simulink model "q3_1"  (R2026a)
settings: Solver=VariableStepAuto  StopTime=1
undefined symbols (not defined in the file): DiscIntNeverNeededParam
libraries: dspstat3 x4, dspfdesign x3, dspmathops x2, dspsrcs4 x1
settings Model: Creator=steve  LastModifiedBy=steve

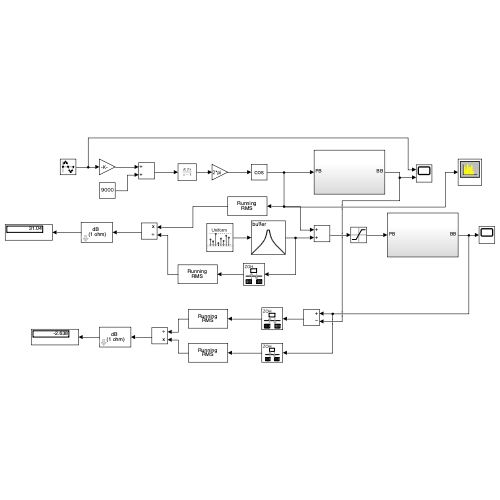
[thumbnail: Simulink's stored preview of the top-level diagram]
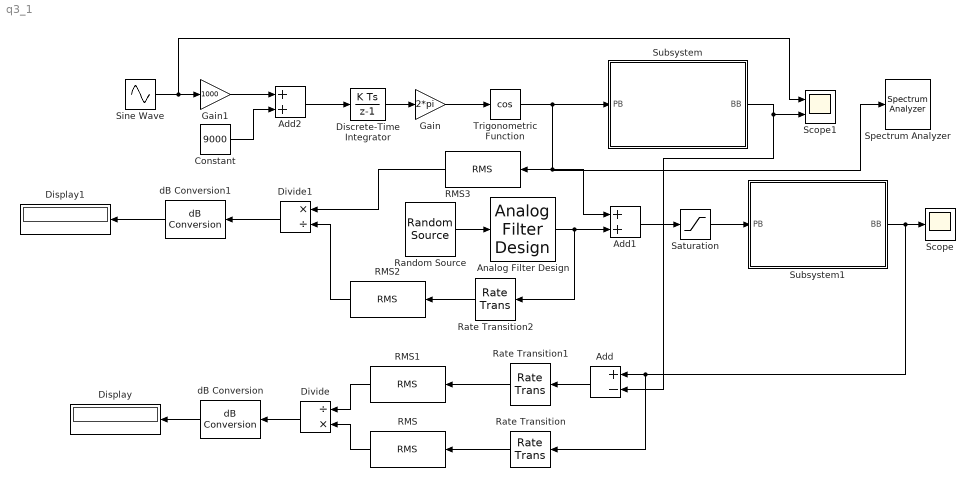
== system q3_1 ==
  Add : Sum  Inputs=+-
  Add1 : Sum
  Add2 : Sum
  Analog Filter Design : dspfdesign/Analog Filter Design  method=Butterworth  filttype=Bandpass  N=8  Wlo=8000*2*pi  Whi=10000*2*pi  Rp=2  Rs=40
  Constant : Constant  Value=9000
  Discrete-Time Integrator : DiscreteIntegrator  SampleTime=1e-5  ICPrevOutput=DiscIntNeverNeededParam  ICPrevScaledInput=DiscIntNeverNeededParam
  Display : Display
  Display1 : Display
  Divide : Product  Inputs=/*
  Divide1 : Product  Inputs=*/
  Gain : Gain  Gain=2*pi
  Gain1 : Gain  Gain=1000
  RMS{,1..3} (4 alike) : dspstat3/RMS  run=on  directionMode=Each column  dimension=1  InputProcessing=Columns as channels (frame based)  reset_popup=None
  Random Source : dspsrcs4/Random Source  SrcType=Gaussian  MinVal=0  MaxVal=1  MeanVal=0  VarVal=1e-2  RepMode=Specify seed  rawSeed=1  IsInherit=off  SampTime=1e-5  SampFrame=1  OutComplex=Real  DataType=double  SimulateUsing=Interpreted execution
  Rate Transition : RateTransition  OutPortSampleTime=1e-5
  Rate Transition1 : RateTransition  OutPortSampleTime=1e-5
  Rate Transition2 : RateTransition  OutPortSampleTime=1e-5
  Saturation : Saturate  UpperLimit=1  LowerLimit=-1
  Scope : Scope
  Scope1 : Scope  NumInputPorts=2
  Sine Wave : Sin  SineType=Sample based  Samples=1000  SampleTime=1e-5
  Spectrum Analyzer : SpectrumAnalyzer  WindowPosition=[1.000000,65.000000,1470.000000,826.000000,]  ScopeFrameLocation=window  WindowInvariantSamplesPerUpdate=on  YLimits=[-89.9778 31.3294]
  Subsystem : Subsystem
  Subsystem1 : Subsystem
  Trigonometric Function : Trigonometry  Operator=cos
  dB Conversion : dspmathops/dB Conversion  dBtype=dB  intype=Amplitude  R=1  fuzz=off
  dB Conversion1 : dspmathops/dB Conversion  dBtype=dB  intype=Amplitude  R=1  fuzz=off
  wires:
  Sine Wave/1 -> Scope1/1, Gain1/1
  Gain1/1 -> Add2/1
  Constant/1 -> Add2/2
  Add2/1 -> Discrete-Time Integrator/1
  Discrete-Time Integrator/1 -> Gain/1
  Gain/1 -> Trigonometric Function/1
  Trigonometric Function/1 -> Add1/1, Spectrum Analyzer/1, RMS3/1, Subsystem/1(PB)
  dB Conversion1/1 -> Display1/1
  Divide1/1 -> dB Conversion1/1
  RMS3/1 -> Divide1/1
  Random Source/1 -> Analog Filter Design/1
  Analog Filter Design/1 -> Rate Transition2/1, Add1/2
  Add1/1 -> Saturation/1
  Saturation/1 -> Subsystem1/1(PB)
  Subsystem1/1(BB) -> Rate Transition/1, Add/1, Scope/1
  RMS2/1 -> Divide1/2
  Rate Transition2/1 -> RMS2/1
  Divide/1 -> dB Conversion/1
  dB Conversion/1 -> Display/1
  Add/1 -> Rate Transition1/1
  RMS1/1 -> Divide/1
  RMS/1 -> Divide/2
  Rate Transition1/1 -> RMS1/1
  Rate Transition/1 -> RMS/1
  Subsystem/1(BB) -> Add/2, Scope1/2

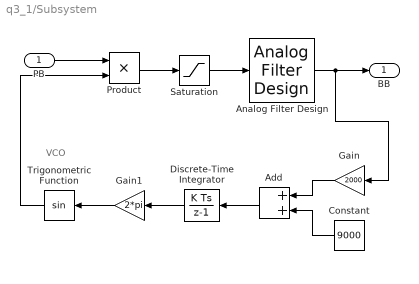
== system q3_1/Subsystem ==
  note: VCO
  PB : Inport
  Add : Sum
  Analog Filter Design : dspfdesign/Analog Filter Design  method=Butterworth  filttype=Lowpass  N=8  Wlo=200*2*pi  Whi=80  Rp=2  Rs=40
  Constant : Constant  Value=9000
  Discrete-Time Integrator : DiscreteIntegrator  SampleTime=1e-5  ICPrevOutput=DiscIntNeverNeededParam  ICPrevScaledInput=DiscIntNeverNeededParam
  Gain : Gain  Gain=2000
  Gain1 : Gain  Gain=2*pi
  Product : Product
  Saturation : Saturate
  Trigonometric Function : Trigonometry
  BB : Outport
  wires:
  Discrete-Time Integrator/1 -> Gain1/1
  PB/1 -> Product/1
  Add/1 -> Discrete-Time Integrator/1
  Analog Filter Design/1 -> BB/1, Gain/1
  Constant/1 -> Add/2
  Saturation/1 -> Analog Filter Design/1
  Gain1/1 -> Trigonometric Function/1
  Gain/1 -> Add/1
  Trigonometric Function/1 -> Product/2
  Product/1 -> Saturation/1

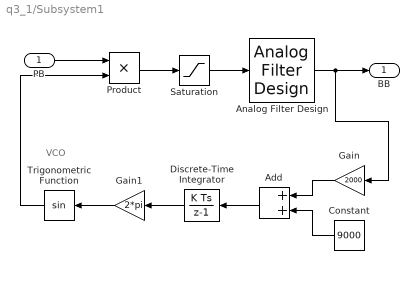
== system q3_1/Subsystem1 ==
  note: VCO
  PB : Inport
  Add : Sum
  Analog Filter Design : dspfdesign/Analog Filter Design  method=Butterworth  filttype=Lowpass  N=8  Wlo=200*2*pi  Whi=80  Rp=2  Rs=40
  Constant : Constant  Value=9000
  Discrete-Time Integrator : DiscreteIntegrator  SampleTime=1e-5  ICPrevOutput=DiscIntNeverNeededParam  ICPrevScaledInput=DiscIntNeverNeededParam
  Gain : Gain  Gain=2000
  Gain1 : Gain  Gain=2*pi
  Product : Product
  Saturation : Saturate
  Trigonometric Function : Trigonometry
  BB : Outport
  wires:
  Discrete-Time Integrator/1 -> Gain1/1
  PB/1 -> Product/1
  Add/1 -> Discrete-Time Integrator/1
  Analog Filter Design/1 -> BB/1, Gain/1
  Constant/1 -> Add/2
  Saturation/1 -> Analog Filter Design/1
  Gain1/1 -> Trigonometric Function/1
  Gain/1 -> Add/1
  Trigonometric Function/1 -> Product/2
  Product/1 -> Saturation/1
